simulink model "BPSK_Model"  (R2024b)
settings: Solver=VariableStepAuto  StartTime=0.0  StopTime=136  RelTol=1e-3
values from neighbouring files (symbols this model uses):
  bitMatrix = zeros(nSats, maxLen)    [bitMatrixAllocation.m]
libraries: dspsrcs4 x1
settings Model: Creator=navra  LastModifiedBy=navra

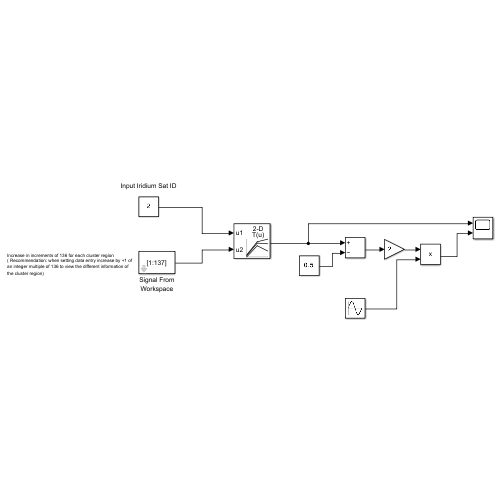
[thumbnail: Simulink's stored preview of the top-level diagram]
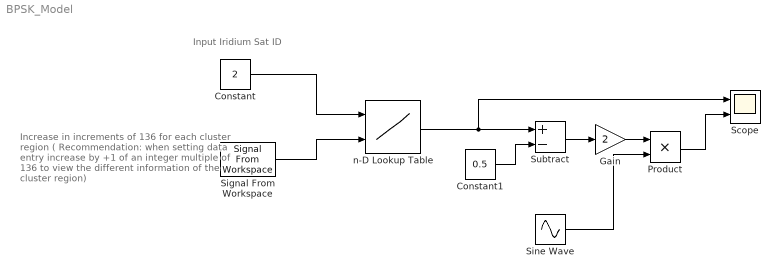
== system BPSK_Model ==
  note: Increase in increments of 136 for each cluster region
      | ( Recommendation: when setting data entry increase by +1 of an integer multiple of 136 to view the different information of the cluster region)
  note: Input Iridium Sat ID
  Constant : Constant  Value=2
  Constant1 : Constant  Value=0.5
  Gain : Gain  Gain=2
  Product : Product
  Scope : Scope  NumInputPorts=2
  Signal From Workspace : dspsrcs4/Signal From Workspace  X=[1:137]  Ts=5  nsamps=1  OutputAfterFinalValue=Setting to zero  ignoreOrWarnInputAndFrameLengths=off  OutputFrames=off
  Sine Wave : Sin  Frequency=2*pi/5  SampleTime=0
  Subtract : Sum  Inputs=+-
  n-D Lookup Table : Lookup_n-D  BreakpointsForDimension1=[1:66]  BreakpointsForDimension2=[1:73002]  Table=bitMatrix  RndMeth=Simplest
      settings: InputPortMap=u0,u1
  wires:
  Constant/1 -> n-D Lookup Table/1
  Signal From Workspace/1 -> n-D Lookup Table/2
  Constant1/1 -> Subtract/2
  Subtract/1 -> Gain/1
  Sine Wave/1 -> Product/2
  Gain/1 -> Product/1
  Product/1 -> Scope/2
  n-D Lookup Table/1 -> Subtract/1, Scope/1
